simulink model "Add"  (R2021a)
settings: Solver=VariableStepAuto  StartTime=0.0  StopTime=10.0  RelTol=1e-3
settings Model: Creator=User  LastModifiedBy=User

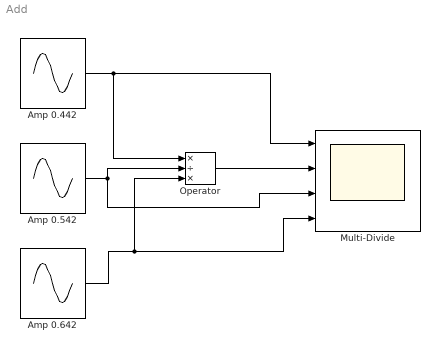
== system Add ==
  Amp 0.442 : Sin  Amplitude=0.442  SampleTime=0
  Amp 0.542 : Sin  Amplitude=0.542  SampleTime=0
  Amp 0.642 : Sin  Amplitude=0.642  SampleTime=0
  Multi-Divide : Scope  NumInputPorts=4
  Operator : Product  Inputs=*/*
  wires:
  Amp 0.442/1 -> Operator/1, Multi-Divide/1
  Amp 0.642/1 -> Operator/3, Multi-Divide/4
  Operator/1 -> Multi-Divide/2
  Amp 0.542/1 -> Operator/2, Multi-Divide/3
